simulink model "controllers_c_model"  (R2019b)
settings: Solver=FixedStepDiscrete  StartTime=0.0  StopTime=10.0  FixedStep=Ts  RelTol=1e-3
PreLoadFcn:
  | Ts = 0.01
InitFcn:
  | Ts = 0.01
  | mex controller.c
settings Model: Creator=Kamran  LastModifiedBy=Kamran

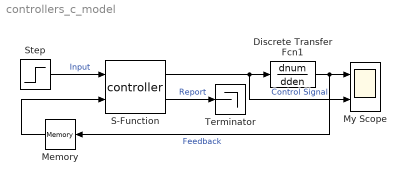
== system controllers_c_model ==
  Discrete Transfer Fcn1 : DiscreteTransferFcn  Numerator=dnum  Denominator=dden  mask{num=1, den=[1 1], ts=Ts}
      mask prompts: num "Numerator"; den "Denominator"; ts "Sampling Time"
      mask help: A simple mask over a discrete transfer function with normal understandable Laplace form inputs.
      mask init:
      | sys = c2d(tf(num, den), ts, 'Tustin');
      | dnum = sys.Numerator{1};
      | dden = sys.Denominator{1};
      mask Display: disp('plant')
  Memory : Memory
  My Scope : Scope  NumInputPorts=2
  S-Function : S-Function  FunctionName=controller  Parameters=Ts  SFunctionDeploymentMode=off  EnableBusSupport=off
  Step : Step  SampleTime=Ts
  Terminator : Terminator
  wires:
  Discrete Transfer Fcn1/1 -> Memory/1, My Scope/1  "Feedback"
  Step/1 -> S-Function/1  "Input"
  S-Function/2 -> Terminator/1  "Report"
  S-Function/1 -> Discrete Transfer Fcn1/1, My Scope/2  "Control Signal"
  Memory/1 -> S-Function/2
